simulink subsystem "ChillerDummy"  (R2024b)
settings: Solver=VariableStepAuto  StartTime=0.0  StopTime=10.0  RelTol=1e-3
undefined symbols (not defined in the file or in its folder): chiller
libraries: fl_lib x3, nesl_utility x1
Description:
  | Minimal chiller stub with fixed electrical load. Draws constant current (P_max/V_nom) when chiller is active (cmdChillerByp=0). Coolant passes through with no heat exchange. Same port interface as Chiller.slx.
settings Model: Creator=jjha  LastModifiedBy=jjha

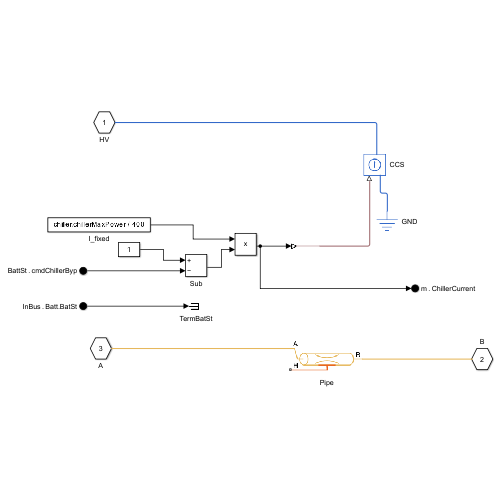
[thumbnail: Simulink's stored preview of the top-level diagram]
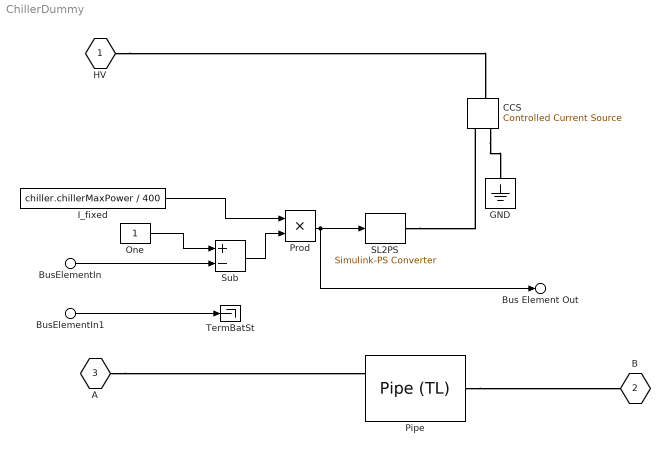
== system ChillerDummy ==
  BusElementIn1 : Inport  PortName=InBus  Element=Batt.BatSt
  BusElementIn : Inport  Port=2  PortName=BattSt  Element=cmdChillerByp
  CCS : fl_lib/Electrical/Electrical Sources/Controlled Current Source
  GND : fl_lib/Electrical/Electrical Elements/Electrical Reference
  I_fixed : Constant  Value=chiller.chillerMaxPower / 400
  One : Constant
  Pipe : fl_lib/Thermal Liquid/Elements/Pipe (TL)  length=5 m  area=0.01 m^2  Dh=0.1128 m  length_add=1 m  roughness=15e-6 m  Re_lam=2000  Re_tur=4000  shape_factor=64  Nu_lam=3.66  dynamic_compressibility=true  inertia=false  p0=0.101325 MPa  T0=293.15 K  mdot0=0 kg/s
  Prod : Product
  SL2PS : nesl_utility/Simulink-PS Converter  PhysicalDomain=network_engine_domain  SubClassName=ps_input  LeftPortType=input  RightPortType=output  PseudoPeriodic=off  Frequencies=[]  NoiseDistribution=none  NoiseParameters=[]  Unit=1  AffineConversion=off  FilteringAndDerivatives=provide  SimscapeFilterOrder=1  InputFilterTimeConstant=0.001  UdotUserProvided=0
  Sub : Sum  Inputs=+-
  TermBatSt : Terminator
  HV : PMIOPort  Side=Left
  B : PMIOPort  Port=2  Side=Right
  A : PMIOPort  Port=3  Side=Left
  Bus Element Out : Outport  PortName=m  Element=ChillerCurrent
  wires:
  BusElementIn1/1 -> TermBatSt/1
  One/1 -> Sub/1
  BusElementIn/1 -> Sub/2
  I_fixed/1 -> Prod/1
  Sub/1 -> Prod/2
  Prod/1 -> Bus Element Out/1, SL2PS/1
  connections:
  CCS/RConn2 -- GND/LConn1
  HV/RConn1 -- CCS/LConn1
  A/RConn1 -- Pipe/LConn1
  Pipe/RConn1 -- B/RConn1
  SL2PS/RConn1 -- CCS/RConn1
